simulink model "KeylessEntryArchitecture"  (R2024a)
settings: Solver=VariableStepAuto  StartTime=0.0  StopTime=10.0  RelTol=1e-3
settings Model: DataDictionary=Interfaces.sldd  Creator=The MathWorks, Inc.  LastModifiedBy=The MathWorks, Inc.
settings SolverCC: AlgebraicLoopSolver=TrustRegion
settings DebuggingCC: UnconnectedInputMsg=warning  UnconnectedOutputMsg=warning  UnconnectedLineMsg=warning  SymbolicDimsDataTypeCodeGenerationDiagnostic=none
settings ModelReferenceCC: EnableRefExpFcnMdlSchedulingChecks=on
settings RTWCC: GPUComputeCapability=3.5  DLArmComputeVersion=19.05

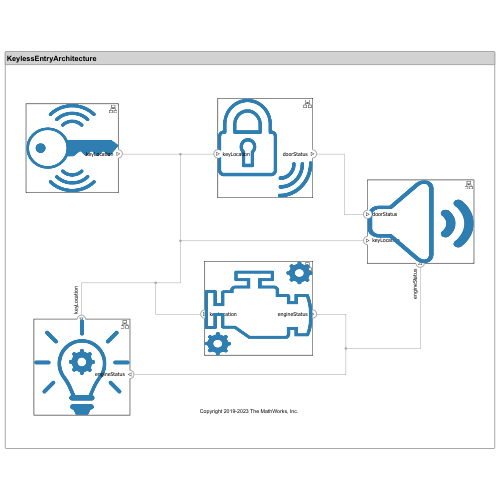
[thumbnail: Simulink's stored preview of the top-level diagram]
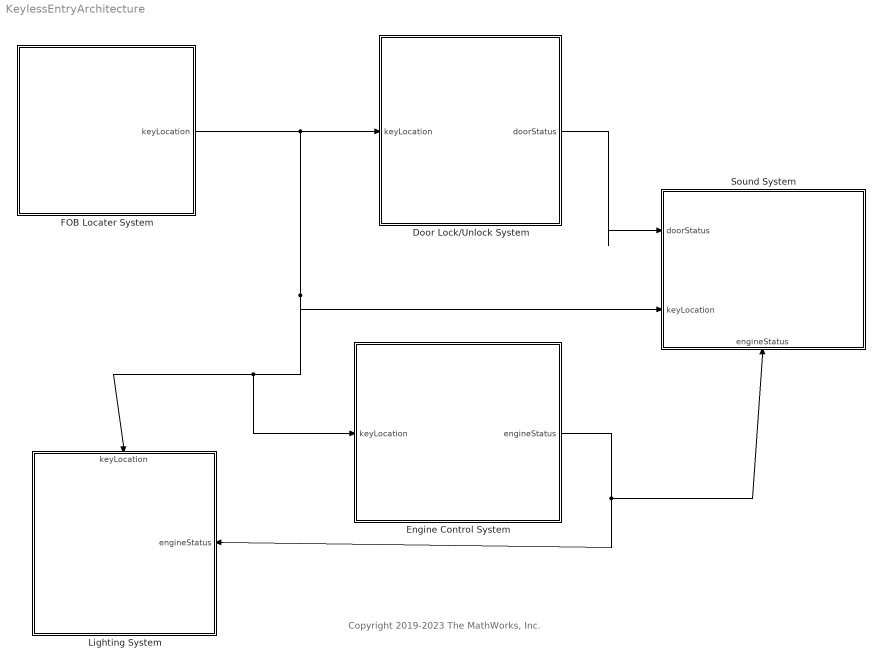
== system KeylessEntryArchitecture ==
  note: Copyright 2019-2023 The MathWorks, Inc.
  Door Lock/Unlock System : Subsystem
      settings: PortSchema="{\"entries\":[{\"content\":{\"headerSize\":26,\"margin\":15,\"minimumSpacing\":25,\"sides\":[{\"content\":{\"connectorIds\":[\"In1\"]},\"type\":\"ConnectorPlacement.EquallySpacedRectSide\",\"uuid\":\"159ee682-9fed-4fbb-9d94-5dba31d2910e\"},{\"content\":{\"connectorIds\":[\"Out1\"],\"side\":\"RIGHT\"},\"type\":\"ConnectorPlacement.EquallySpacedRectSide\",\"uuid\":\"29b28cc0-b170-4369-a93a-656923dab01a\"},{\"content\":{\"connectorIds\":[],\"side\":\"TOP\"},\"type\":\"ConnectorPlacement.EquallySpacedRectSide\",\"uuid\":\"ccfc0ebb-e385-4049-95f8-9f41f6dbc5fa\"}]},\"type\":\"ConnectorPlacement.EquallySpacedConnector\",\"uuid\":\"edbc9e1e-b6af-4ee7-9cbe-c6e12d5af40d\"}],\"packageUris\":[\"http://schema.mathworks.com/mf0/Connector/19700101\"],\"version\":\"1.0\"}"
      mask Display: image('door_lock_icon.png');
  Engine Control System : Subsystem
      settings: PortSchema="{\"entries\":[{\"content\":{\"headerSize\":26,\"margin\":15,\"minimumSpacing\":25,\"sides\":[{\"content\":{\"connectorIds\":[\"In1\"]},\"type\":\"ConnectorPlacement.EquallySpacedRectSide\",\"uuid\":\"159ee682-9fed-4fbb-9d94-5dba31d2910e\"},{\"content\":{\"connectorIds\":[\"Out1\"],\"side\":\"RIGHT\"},\"type\":\"ConnectorPlacement.EquallySpacedRectSide\",\"uuid\":\"29b28cc0-b170-4369-a93a-656923dab01a\"},{\"content\":{\"connectorIds\":[],\"side\":\"TOP\"},\"type\":\"ConnectorPlacement.EquallySpacedRectSide\",\"uuid\":\"ccfc0ebb-e385-4049-95f8-9f41f6dbc5fa\"}]},\"type\":\"ConnectorPlacement.EquallySpacedConnector\",\"uuid\":\"edbc9e1e-b6af-4ee7-9cbe-c6e12d5af40d\"}],\"packageUris\":[\"http://schema.mathworks.com/mf0/Connector/19700101\"],\"version\":\"1.0\"}"
      mask Display: image('engine_control_icon.png');
  FOB Locater System : Subsystem
      settings: PortSchema="{\"entries\":[{\"content\":{\"headerSize\":26,\"margin\":15,\"minimumSpacing\":25,\"sides\":[{\"content\":{\"connectorIds\":[]},\"type\":\"ConnectorPlacement.EquallySpacedRectSide\",\"uuid\":\"159ee682-9fed-4fbb-9d94-5dba31d2910e\"},{\"content\":{\"connectorIds\":[\"Out1\"],\"side\":\"RIGHT\"},\"type\":\"ConnectorPlacement.EquallySpacedRectSide\",\"uuid\":\"29b28cc0-b170-4369-a93a-656923dab01a\"},{\"content\":{\"connectorIds\":[],\"side\":\"TOP\"},\"type\":\"ConnectorPlacement.EquallySpacedRectSide\",\"uuid\":\"ccfc0ebb-e385-4049-95f8-9f41f6dbc5fa\"}]},\"type\":\"ConnectorPlacement.EquallySpacedConnector\",\"uuid\":\"edbc9e1e-b6af-4ee7-9cbe-c6e12d5af40d\"}],\"packageUris\":[\"http://schema.mathworks.com/mf0/Connector/19700101\"],\"version\":\"1.0\"}"
      mask Display: image('fob_locator_icon.png');
  Lighting System : Subsystem
      settings: PortSchema="{\"entries\":[{\"content\":{\"headerSize\":26,\"margin\":15,\"minimumSpacing\":25,\"sides\":[{\"content\":{\"connectorIds\":[]},\"type\":\"ConnectorPlacement.EquallySpacedRectSide\",\"uuid\":\"159ee682-9fed-4fbb-9d94-5dba31d2910e\"},{\"content\":{\"connectorIds\":[\"In2\"],\"side\":\"RIGHT\"},\"type\":\"ConnectorPlacement.EquallySpacedRectSide\",\"uuid\":\"29b28cc0-b170-4369-a93a-656923dab01a\"},{\"content\":{\"connectorIds\":[\"In1\"],\"side\":\"TOP\"},\"type\":\"ConnectorPlacement.EquallySpacedRectSide\",\"uuid\":\"ccfc0ebb-e385-4049-95f8-9f41f6dbc5fa\"}]},\"type\":\"ConnectorPlacement.EquallySpacedConnector\",\"uuid\":\"edbc9e1e-b6af-4ee7-9cbe-c6e12d5af40d\"}],\"packageUris\":[\"http://schema.mathworks.com/mf0/Connector/19700101\"],\"version\":\"1.0\"}"
      mask Display: image('lighting_system_icon.png');
  Sound System : Subsystem
      settings: PortSchema="{\"entries\":[{\"content\":{\"headerSize\":26,\"margin\":15,\"minimumSpacing\":25,\"sides\":[{\"content\":{\"connectorIds\":[\"In3\",\"In2\"]},\"type\":\"ConnectorPlacement.EquallySpacedRectSide\",\"uuid\":\"159ee682-9fed-4fbb-9d94-5dba31d2910e\"},{\"content\":{\"connectorIds\":[],\"side\":\"RIGHT\"},\"type\":\"ConnectorPlacement.EquallySpacedRectSide\",\"uuid\":\"29b28cc0-b170-4369-a93a-656923dab01a\"},{\"content\":{\"connectorIds\":[],\"side\":\"TOP\"},\"type\":\"ConnectorPlacement.EquallySpacedRectSide\",\"uuid\":\"ccfc0ebb-e385-4049-95f8-9f41f6dbc5fa\"},{\"content\":{\"connectorIds\":[\"In1\"],\"side\":\"BOTTOM\"},\"type\":\"ConnectorPlacement.EquallySpacedRectSide\",\"uuid\":\"874e8f25-aa17-4249-8800-ee0df902b395\"}]},\"type\":\"ConnectorPlacement.EquallySpacedConnector\",\"uuid\":\"edbc9e1e-b6af-4ee7-9cbe-c6e12d5af40d\"}],\"packageUris\":[\"http://schema.mathworks.com/mf0/Connector/19700101\"],\"version\":\"1.0\"}"
      mask Display: image('sound_system_icon.png');
  wires:
  FOB Locater System/1(keyLocation) -> Door Lock/Unlock System/1(keyLocation), Lighting System/1(keyLocation), Engine Control System/1(keyLocation), Sound System/2(keyLocation)
  Door Lock/Unlock System/1(doorStatus) -> Sound System/3(doorStatus)
  Engine Control System/1(engineStatus) -> Lighting System/2(engineStatus), Sound System/1(engineStatus)

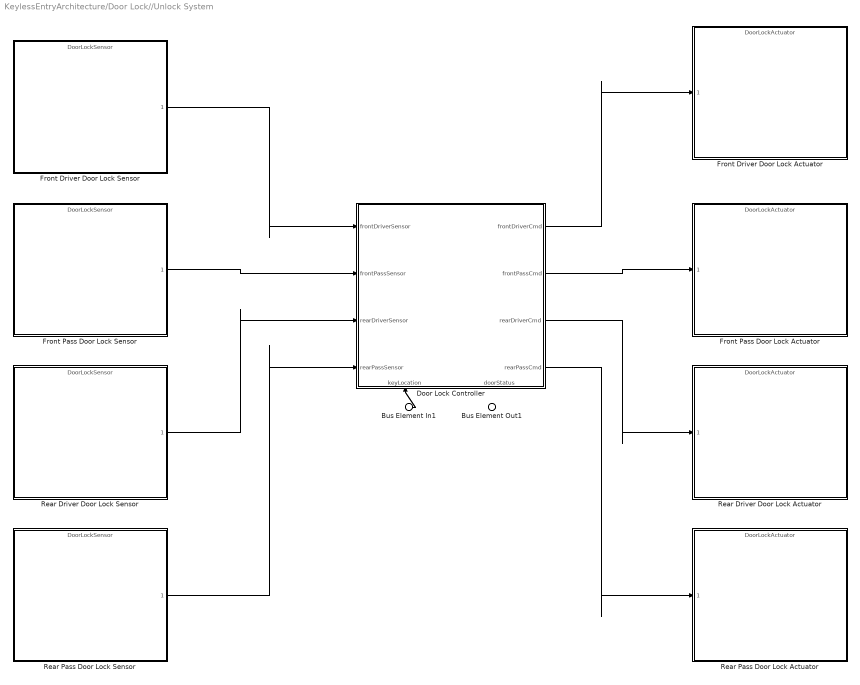
== system KeylessEntryArchitecture/Door Lock//Unlock System ==
  Bus Element In1 : Inport  PortName=keyLocation
  Door Lock Controller : Subsystem
      settings: PortSchema="{\"entries\":[{\"content\":{\"headerSize\":26,\"margin\":15,\"minimumSpacing\":25,\"sides\":[{\"content\":{\"connectorIds\":[\"In2\",\"In3\",\"In4\",\"In5\"]},\"type\":\"ConnectorPlacement.EquallySpacedRectSide\",\"uuid\":\"a0f82e88-5275-4bb9-87fe-a49bf19782cf\"},{\"content\":{\"connectorIds\":[\"Out1\",\"Out3\",\"Out4\",\"Out5\"],\"side\":\"RIGHT\"},\"type\":\"ConnectorPlacement.EquallySpacedRectSide\",\"uuid\":\"4b3945c4-3891-41a7-b741-bb467a4ccb5a\"},{\"content\":{\"connectorIds\":[],\"side\":\"TOP\"},\"type\":\"ConnectorPlacement.EquallySpacedRectSide\",\"uuid\":\"042b1b4e-e1cf-4b0e-a9d9-106bb99a7cf5\"},{\"content\":{\"connectorIds\":[\"In1\",\"Out2\"],\"side\":\"BOTTOM\"},\"type\":\"ConnectorPlacement.EquallySpacedRectSide\",\"uuid\":\"6aa53690-4f36-48a3-9490-70419d307c63\"}]},\"type\":\"ConnectorPlacement.EquallySpacedConnector\",\"uuid\":\"79d888da-39cf-4e1d-aa7b-1e8818e96d62\"}],\"packageUris\":[\"http://schema.mathworks.com/mf0/Connector/19700101\"],\"version\":\"1.0\"}"
  Front Driver Door Lock Actuator : ModelReference  ModelNameDialog=DoorLockActuator  SimulationMode=Normal  ModelReferenceVersion=8.5
      settings: PortSchema="{\"entries\":[{\"content\":{\"headerSize\":38,\"margin\":15,\"minimumSpacing\":25,\"sides\":[{\"content\":{\"connectorIds\":[\"In1\"]},\"type\":\"ConnectorPlacement.EquallySpacedRectSide\",\"uuid\":\"a0f82e88-5275-4bb9-87fe-a49bf19782cf\"},{\"content\":{\"connectorIds\":[],\"side\":\"RIGHT\"},\"type\":\"ConnectorPlacement.EquallySpacedRectSide\",\"uuid\":\"4b3945c4-3891-41a7-b741-bb467a4ccb5a\"},{\"content\":{\"connectorIds\":[],\"side\":\"TOP\"},\"type\":\"ConnectorPlacement.EquallySpacedRectSide\",\"uuid\":\"042b1b4e-e1cf-4b0e-a9d9-106bb99a7cf5\"}]},\"type\":\"ConnectorPlacement.EquallySpacedConnector\",\"uuid\":\"79d888da-39cf-4e1d-aa7b-1e8818e96d62\"}],\"packageUris\":[\"http://schema.mathworks.com/mf0/Connector/19700101\"],\"version\":\"1.0\"}"
  Front Driver Door Lock Sensor : ModelReference  ModelNameDialog=DoorLockSensor  SimulationMode=Normal  ModelReferenceVersion=8.5
      settings: PortSchema="{\"entries\":[{\"content\":{\"headerSize\":38,\"margin\":15,\"minimumSpacing\":25,\"sides\":[{\"content\":{\"connectorIds\":[]},\"type\":\"ConnectorPlacement.EquallySpacedRectSide\",\"uuid\":\"a0f82e88-5275-4bb9-87fe-a49bf19782cf\"},{\"content\":{\"connectorIds\":[\"Out1\"],\"side\":\"RIGHT\"},\"type\":\"ConnectorPlacement.EquallySpacedRectSide\",\"uuid\":\"4b3945c4-3891-41a7-b741-bb467a4ccb5a\"},{\"content\":{\"connectorIds\":[],\"side\":\"TOP\"},\"type\":\"ConnectorPlacement.EquallySpacedRectSide\",\"uuid\":\"042b1b4e-e1cf-4b0e-a9d9-106bb99a7cf5\"}]},\"type\":\"ConnectorPlacement.EquallySpacedConnector\",\"uuid\":\"79d888da-39cf-4e1d-aa7b-1e8818e96d62\"}],\"packageUris\":[\"http://schema.mathworks.com/mf0/Connector/19700101\"],\"version\":\"1.0\"}"
  Front Pass Door Lock Actuator : ModelReference  ModelNameDialog=DoorLockActuator  SimulationMode=Normal  ModelReferenceVersion=8.5
      settings: PortSchema="{\"entries\":[{\"content\":{\"headerSize\":38,\"margin\":15,\"minimumSpacing\":25,\"sides\":[{\"content\":{\"connectorIds\":[\"In1\"]},\"type\":\"ConnectorPlacement.EquallySpacedRectSide\",\"uuid\":\"a0f82e88-5275-4bb9-87fe-a49bf19782cf\"},{\"content\":{\"connectorIds\":[],\"side\":\"RIGHT\"},\"type\":\"ConnectorPlacement.EquallySpacedRectSide\",\"uuid\":\"4b3945c4-3891-41a7-b741-bb467a4ccb5a\"},{\"content\":{\"connectorIds\":[],\"side\":\"TOP\"},\"type\":\"ConnectorPlacement.EquallySpacedRectSide\",\"uuid\":\"042b1b4e-e1cf-4b0e-a9d9-106bb99a7cf5\"}]},\"type\":\"ConnectorPlacement.EquallySpacedConnector\",\"uuid\":\"79d888da-39cf-4e1d-aa7b-1e8818e96d62\"}],\"packageUris\":[\"http://schema.mathworks.com/mf0/Connector/19700101\"],\"version\":\"1.0\"}"
  Front Pass Door Lock Sensor : ModelReference  ModelNameDialog=DoorLockSensor  SimulationMode=Normal  ModelReferenceVersion=8.5
      settings: PortSchema="{\"entries\":[{\"content\":{\"headerSize\":38,\"margin\":15,\"minimumSpacing\":25,\"sides\":[{\"content\":{\"connectorIds\":[]},\"type\":\"ConnectorPlacement.EquallySpacedRectSide\",\"uuid\":\"a0f82e88-5275-4bb9-87fe-a49bf19782cf\"},{\"content\":{\"connectorIds\":[\"Out1\"],\"side\":\"RIGHT\"},\"type\":\"ConnectorPlacement.EquallySpacedRectSide\",\"uuid\":\"4b3945c4-3891-41a7-b741-bb467a4ccb5a\"},{\"content\":{\"connectorIds\":[],\"side\":\"TOP\"},\"type\":\"ConnectorPlacement.EquallySpacedRectSide\",\"uuid\":\"042b1b4e-e1cf-4b0e-a9d9-106bb99a7cf5\"}]},\"type\":\"ConnectorPlacement.EquallySpacedConnector\",\"uuid\":\"79d888da-39cf-4e1d-aa7b-1e8818e96d62\"}],\"packageUris\":[\"http://schema.mathworks.com/mf0/Connector/19700101\"],\"version\":\"1.0\"}"
  Rear Driver Door Lock Actuator : ModelReference  ModelNameDialog=DoorLockActuator  SimulationMode=Normal  ModelReferenceVersion=8.5
      settings: PortSchema="{\"entries\":[{\"content\":{\"headerSize\":38,\"margin\":15,\"minimumSpacing\":25,\"sides\":[{\"content\":{\"connectorIds\":[\"In1\"]},\"type\":\"ConnectorPlacement.EquallySpacedRectSide\",\"uuid\":\"a0f82e88-5275-4bb9-87fe-a49bf19782cf\"},{\"content\":{\"connectorIds\":[],\"side\":\"RIGHT\"},\"type\":\"ConnectorPlacement.EquallySpacedRectSide\",\"uuid\":\"4b3945c4-3891-41a7-b741-bb467a4ccb5a\"},{\"content\":{\"connectorIds\":[],\"side\":\"TOP\"},\"type\":\"ConnectorPlacement.EquallySpacedRectSide\",\"uuid\":\"042b1b4e-e1cf-4b0e-a9d9-106bb99a7cf5\"}]},\"type\":\"ConnectorPlacement.EquallySpacedConnector\",\"uuid\":\"79d888da-39cf-4e1d-aa7b-1e8818e96d62\"}],\"packageUris\":[\"http://schema.mathworks.com/mf0/Connector/19700101\"],\"version\":\"1.0\"}"
  Rear Driver Door Lock Sensor : ModelReference  ModelNameDialog=DoorLockSensor  SimulationMode=Normal  ModelReferenceVersion=8.5
      settings: PortSchema="{\"entries\":[{\"content\":{\"headerSize\":38,\"margin\":15,\"minimumSpacing\":25,\"sides\":[{\"content\":{\"connectorIds\":[]},\"type\":\"ConnectorPlacement.EquallySpacedRectSide\",\"uuid\":\"a0f82e88-5275-4bb9-87fe-a49bf19782cf\"},{\"content\":{\"connectorIds\":[\"Out1\"],\"side\":\"RIGHT\"},\"type\":\"ConnectorPlacement.EquallySpacedRectSide\",\"uuid\":\"4b3945c4-3891-41a7-b741-bb467a4ccb5a\"},{\"content\":{\"connectorIds\":[],\"side\":\"TOP\"},\"type\":\"ConnectorPlacement.EquallySpacedRectSide\",\"uuid\":\"042b1b4e-e1cf-4b0e-a9d9-106bb99a7cf5\"}]},\"type\":\"ConnectorPlacement.EquallySpacedConnector\",\"uuid\":\"79d888da-39cf-4e1d-aa7b-1e8818e96d62\"}],\"packageUris\":[\"http://schema.mathworks.com/mf0/Connector/19700101\"],\"version\":\"1.0\"}"
  Rear Pass Door Lock Actuator : ModelReference  ModelNameDialog=DoorLockActuator  SimulationMode=Normal  ModelReferenceVersion=8.5
      settings: PortSchema="{\"entries\":[{\"content\":{\"headerSize\":38,\"margin\":15,\"minimumSpacing\":25,\"sides\":[{\"content\":{\"connectorIds\":[\"In1\"]},\"type\":\"ConnectorPlacement.EquallySpacedRectSide\",\"uuid\":\"a0f82e88-5275-4bb9-87fe-a49bf19782cf\"},{\"content\":{\"connectorIds\":[],\"side\":\"RIGHT\"},\"type\":\"ConnectorPlacement.EquallySpacedRectSide\",\"uuid\":\"4b3945c4-3891-41a7-b741-bb467a4ccb5a\"},{\"content\":{\"connectorIds\":[],\"side\":\"TOP\"},\"type\":\"ConnectorPlacement.EquallySpacedRectSide\",\"uuid\":\"042b1b4e-e1cf-4b0e-a9d9-106bb99a7cf5\"}]},\"type\":\"ConnectorPlacement.EquallySpacedConnector\",\"uuid\":\"79d888da-39cf-4e1d-aa7b-1e8818e96d62\"}],\"packageUris\":[\"http://schema.mathworks.com/mf0/Connector/19700101\"],\"version\":\"1.0\"}"
  Rear Pass Door Lock Sensor : ModelReference  ModelNameDialog=DoorLockSensor  SimulationMode=Normal  ModelReferenceVersion=8.5
      settings: PortSchema="{\"entries\":[{\"content\":{\"headerSize\":38,\"margin\":15,\"minimumSpacing\":25,\"sides\":[{\"content\":{\"connectorIds\":[]},\"type\":\"ConnectorPlacement.EquallySpacedRectSide\",\"uuid\":\"a0f82e88-5275-4bb9-87fe-a49bf19782cf\"},{\"content\":{\"connectorIds\":[\"Out1\"],\"side\":\"RIGHT\"},\"type\":\"ConnectorPlacement.EquallySpacedRectSide\",\"uuid\":\"4b3945c4-3891-41a7-b741-bb467a4ccb5a\"},{\"content\":{\"connectorIds\":[],\"side\":\"TOP\"},\"type\":\"ConnectorPlacement.EquallySpacedRectSide\",\"uuid\":\"042b1b4e-e1cf-4b0e-a9d9-106bb99a7cf5\"}]},\"type\":\"ConnectorPlacement.EquallySpacedConnector\",\"uuid\":\"79d888da-39cf-4e1d-aa7b-1e8818e96d62\"}],\"packageUris\":[\"http://schema.mathworks.com/mf0/Connector/19700101\"],\"version\":\"1.0\"}"
  Bus Element Out1 : Outport  PortName=doorStatus
  wires:
  Front Driver Door Lock Sensor/1 -> Door Lock Controller/2(frontDriverSensor)
  Front Pass Door Lock Sensor/1 -> Door Lock Controller/3(frontPassSensor)
  Rear Driver Door Lock Sensor/1 -> Door Lock Controller/4(rearDriverSensor)
  Rear Pass Door Lock Sensor/1 -> Door Lock Controller/5(rearPassSensor)
  Door Lock Controller/1(frontDriverCmd) -> Front Driver Door Lock Actuator/1
  Door Lock Controller/3(frontPassCmd) -> Front Pass Door Lock Actuator/1
  Door Lock Controller/4(rearDriverCmd) -> Rear Driver Door Lock Actuator/1
  Door Lock Controller/5(rearPassCmd) -> Rear Pass Door Lock Actuator/1
  Bus Element In1/1 -> Door Lock Controller/1(keyLocation)

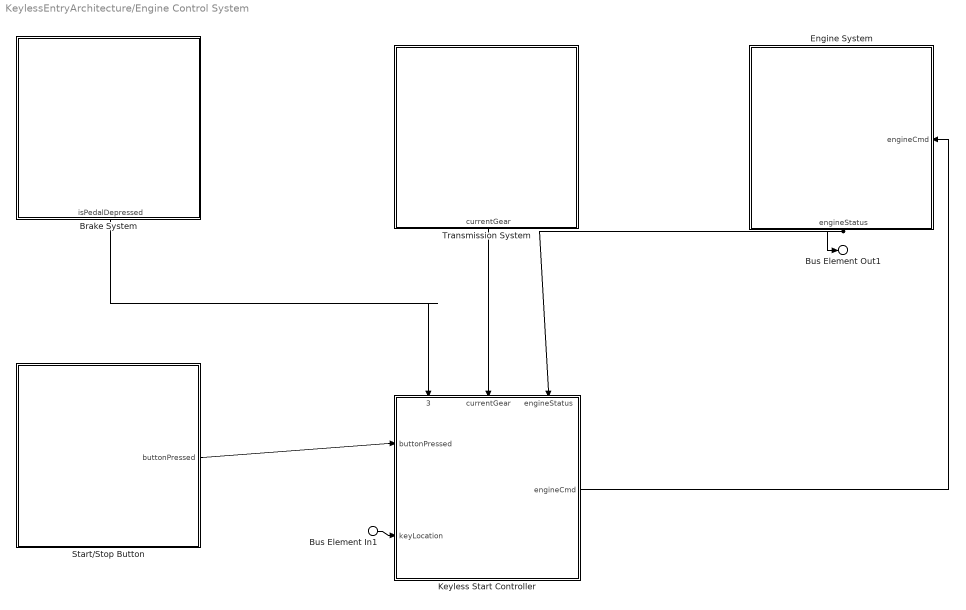
== system KeylessEntryArchitecture/Engine Control System ==
  Bus Element In1 : Inport  PortName=keyLocation
  Brake System : Subsystem
      settings: PortSchema="{\"entries\":[{\"content\":{\"headerSize\":26,\"margin\":15,\"minimumSpacing\":25,\"sides\":[{\"content\":{\"connectorIds\":[]},\"type\":\"ConnectorPlacement.EquallySpacedRectSide\",\"uuid\":\"a0f82e88-5275-4bb9-87fe-a49bf19782cf\"},{\"content\":{\"connectorIds\":[],\"side\":\"RIGHT\"},\"type\":\"ConnectorPlacement.EquallySpacedRectSide\",\"uuid\":\"4b3945c4-3891-41a7-b741-bb467a4ccb5a\"},{\"content\":{\"connectorIds\":[],\"side\":\"TOP\"},\"type\":\"ConnectorPlacement.EquallySpacedRectSide\",\"uuid\":\"042b1b4e-e1cf-4b0e-a9d9-106bb99a7cf5\"},{\"content\":{\"connectorIds\":[\"Out1\"],\"side\":\"BOTTOM\"},\"type\":\"ConnectorPlacement.EquallySpacedRectSide\",\"uuid\":\"2c1eff0a-c33a-441c-bf29-8810011e62b1\"}]},\"type\":\"ConnectorPlacement.EquallySpacedConnector\",\"uuid\":\"79d888da-39cf-4e1d-aa7b-1e8818e96d62\"}],\"packageUris\":[\"http://schema.mathworks.com/mf0/Connector/19700101\"],\"version\":\"1.0\"}"
  Engine System : Subsystem
      settings: PortSchema="{\"entries\":[{\"content\":{\"headerSize\":26,\"margin\":15,\"minimumSpacing\":25,\"sides\":[{\"content\":{\"connectorIds\":[]},\"type\":\"ConnectorPlacement.EquallySpacedRectSide\",\"uuid\":\"a0f82e88-5275-4bb9-87fe-a49bf19782cf\"},{\"content\":{\"connectorIds\":[\"In1\"],\"side\":\"RIGHT\"},\"type\":\"ConnectorPlacement.EquallySpacedRectSide\",\"uuid\":\"4b3945c4-3891-41a7-b741-bb467a4ccb5a\"},{\"content\":{\"connectorIds\":[],\"side\":\"TOP\"},\"type\":\"ConnectorPlacement.EquallySpacedRectSide\",\"uuid\":\"042b1b4e-e1cf-4b0e-a9d9-106bb99a7cf5\"},{\"content\":{\"connectorIds\":[\"Out1\"],\"side\":\"BOTTOM\"},\"type\":\"ConnectorPlacement.EquallySpacedRectSide\",\"uuid\":\"0362089f-4f80-4409-9348-df11b302b3ca\"}]},\"type\":\"ConnectorPlacement.EquallySpacedConnector\",\"uuid\":\"79d888da-39cf-4e1d-aa7b-1e8818e96d62\"}],\"packageUris\":[\"http://schema.mathworks.com/mf0/Connector/19700101\"],\"version\":\"1.0\"}"
  Keyless Start Controller : Subsystem
      settings: PortSchema="{\"entries\":[{\"content\":{\"headerSize\":26,\"margin\":15,\"minimumSpacing\":25,\"sides\":[{\"content\":{\"connectorIds\":[\"In1\",\"In2\"]},\"type\":\"ConnectorPlacement.EquallySpacedRectSide\",\"uuid\":\"a0f82e88-5275-4bb9-87fe-a49bf19782cf\"},{\"content\":{\"connectorIds\":[\"Out1\"],\"side\":\"RIGHT\"},\"type\":\"ConnectorPlacement.EquallySpacedRectSide\",\"uuid\":\"4b3945c4-3891-41a7-b741-bb467a4ccb5a\"},{\"content\":{\"connectorIds\":[\"In3\",\"In4\",\"In5\"],\"side\":\"TOP\"},\"type\":\"ConnectorPlacement.EquallySpacedRectSide\",\"uuid\":\"042b1b4e-e1cf-4b0e-a9d9-106bb99a7cf5\"}]},\"type\":\"ConnectorPlacement.EquallySpacedConnector\",\"uuid\":\"79d888da-39cf-4e1d-aa7b-1e8818e96d62\"}],\"packageUris\":[\"http://schema.mathworks.com/mf0/Connector/19700101\"],\"version\":\"1.0\"}"
  Start/Stop Button : Subsystem
      settings: PortSchema="{\"entries\":[{\"content\":{\"headerSize\":26,\"margin\":15,\"minimumSpacing\":25,\"sides\":[{\"content\":{\"connectorIds\":[]},\"type\":\"ConnectorPlacement.EquallySpacedRectSide\",\"uuid\":\"a0f82e88-5275-4bb9-87fe-a49bf19782cf\"},{\"content\":{\"connectorIds\":[\"Out1\"],\"side\":\"RIGHT\"},\"type\":\"ConnectorPlacement.EquallySpacedRectSide\",\"uuid\":\"4b3945c4-3891-41a7-b741-bb467a4ccb5a\"},{\"content\":{\"connectorIds\":[],\"side\":\"TOP\"},\"type\":\"ConnectorPlacement.EquallySpacedRectSide\",\"uuid\":\"042b1b4e-e1cf-4b0e-a9d9-106bb99a7cf5\"}]},\"type\":\"ConnectorPlacement.EquallySpacedConnector\",\"uuid\":\"79d888da-39cf-4e1d-aa7b-1e8818e96d62\"}],\"packageUris\":[\"http://schema.mathworks.com/mf0/Connector/19700101\"],\"version\":\"1.0\"}"
  Transmission System : Subsystem
      settings: PortSchema="{\"entries\":[{\"content\":{\"headerSize\":26,\"margin\":15,\"minimumSpacing\":25,\"sides\":[{\"content\":{\"connectorIds\":[]},\"type\":\"ConnectorPlacement.EquallySpacedRectSide\",\"uuid\":\"a0f82e88-5275-4bb9-87fe-a49bf19782cf\"},{\"content\":{\"connectorIds\":[],\"side\":\"RIGHT\"},\"type\":\"ConnectorPlacement.EquallySpacedRectSide\",\"uuid\":\"4b3945c4-3891-41a7-b741-bb467a4ccb5a\"},{\"content\":{\"connectorIds\":[],\"side\":\"TOP\"},\"type\":\"ConnectorPlacement.EquallySpacedRectSide\",\"uuid\":\"042b1b4e-e1cf-4b0e-a9d9-106bb99a7cf5\"},{\"content\":{\"connectorIds\":[\"Out1\"],\"side\":\"BOTTOM\"},\"type\":\"ConnectorPlacement.EquallySpacedRectSide\",\"uuid\":\"217a1e67-16b0-4a07-be4d-bf369191c717\"}]},\"type\":\"ConnectorPlacement.EquallySpacedConnector\",\"uuid\":\"79d888da-39cf-4e1d-aa7b-1e8818e96d62\"}],\"packageUris\":[\"http://schema.mathworks.com/mf0/Connector/19700101\"],\"version\":\"1.0\"}"
  Bus Element Out1 : Outport  PortName=engineStatus
  wires:
  Brake System/1(isPedalDepressed) -> Keyless Start Controller/3(isPedalDepressed)
  Transmission System/1(currentGear) -> Keyless Start Controller/4(currentGear)
  Engine System/1(engineStatus) -> Keyless Start Controller/5(engineStatus), Bus Element Out1/1
  Start/Stop Button/1(buttonPressed) -> Keyless Start Controller/1(buttonPressed)
  Keyless Start Controller/1(engineCmd) -> Engine System/1(engineCmd)
  Bus Element In1/1 -> Keyless Start Controller/2(keyLocation)

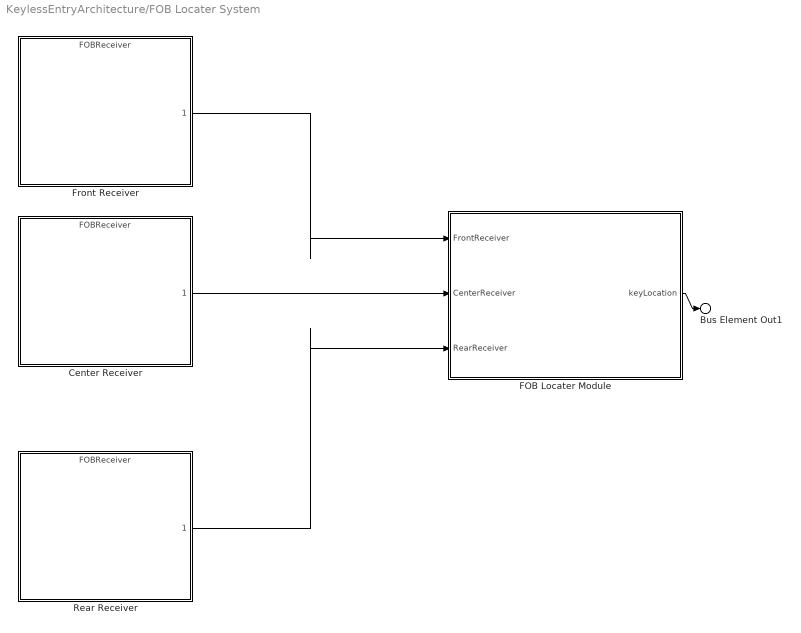
== system KeylessEntryArchitecture/FOB Locater System ==
  Center Receiver : ModelReference  ModelNameDialog=FOBReceiver  SimulationMode=Normal  ModelReferenceVersion=8.6
      settings: PortSchema="{\"entries\":[{\"content\":{\"headerSize\":38,\"margin\":15,\"minimumSpacing\":25,\"sides\":[{\"content\":{\"connectorIds\":[]},\"type\":\"ConnectorPlacement.EquallySpacedRectSide\",\"uuid\":\"a0f82e88-5275-4bb9-87fe-a49bf19782cf\"},{\"content\":{\"connectorIds\":[\"Out1\"],\"side\":\"RIGHT\"},\"type\":\"ConnectorPlacement.EquallySpacedRectSide\",\"uuid\":\"4b3945c4-3891-41a7-b741-bb467a4ccb5a\"},{\"content\":{\"connectorIds\":[],\"side\":\"TOP\"},\"type\":\"ConnectorPlacement.EquallySpacedRectSide\",\"uuid\":\"042b1b4e-e1cf-4b0e-a9d9-106bb99a7cf5\"}]},\"type\":\"ConnectorPlacement.EquallySpacedConnector\",\"uuid\":\"79d888da-39cf-4e1d-aa7b-1e8818e96d62\"}],\"packageUris\":[\"http://schema.mathworks.com/mf0/Connector/19700101\"],\"version\":\"1.0\"}"
  FOB Locater Module : Subsystem
      settings: PortSchema="{\"entries\":[{\"content\":{\"headerSize\":26,\"margin\":15,\"minimumSpacing\":25,\"sides\":[{\"content\":{\"connectorIds\":[\"In1\",\"In2\",\"In3\"]},\"type\":\"ConnectorPlacement.EquallySpacedRectSide\",\"uuid\":\"a0f82e88-5275-4bb9-87fe-a49bf19782cf\"},{\"content\":{\"connectorIds\":[\"Out1\"],\"side\":\"RIGHT\"},\"type\":\"ConnectorPlacement.EquallySpacedRectSide\",\"uuid\":\"4b3945c4-3891-41a7-b741-bb467a4ccb5a\"},{\"content\":{\"connectorIds\":[],\"side\":\"TOP\"},\"type\":\"ConnectorPlacement.EquallySpacedRectSide\",\"uuid\":\"042b1b4e-e1cf-4b0e-a9d9-106bb99a7cf5\"}]},\"type\":\"ConnectorPlacement.EquallySpacedConnector\",\"uuid\":\"79d888da-39cf-4e1d-aa7b-1e8818e96d62\"}],\"packageUris\":[\"http://schema.mathworks.com/mf0/Connector/19700101\"],\"version\":\"1.0\"}"
  Front Receiver : ModelReference  ModelNameDialog=FOBReceiver  SimulationMode=Normal  ModelReferenceVersion=8.6
      settings: PortSchema="{\"entries\":[{\"content\":{\"headerSize\":38,\"margin\":15,\"minimumSpacing\":25,\"sides\":[{\"content\":{\"connectorIds\":[]},\"type\":\"ConnectorPlacement.EquallySpacedRectSide\",\"uuid\":\"a0f82e88-5275-4bb9-87fe-a49bf19782cf\"},{\"content\":{\"connectorIds\":[\"Out1\"],\"side\":\"RIGHT\"},\"type\":\"ConnectorPlacement.EquallySpacedRectSide\",\"uuid\":\"4b3945c4-3891-41a7-b741-bb467a4ccb5a\"},{\"content\":{\"connectorIds\":[],\"side\":\"TOP\"},\"type\":\"ConnectorPlacement.EquallySpacedRectSide\",\"uuid\":\"042b1b4e-e1cf-4b0e-a9d9-106bb99a7cf5\"}]},\"type\":\"ConnectorPlacement.EquallySpacedConnector\",\"uuid\":\"79d888da-39cf-4e1d-aa7b-1e8818e96d62\"}],\"packageUris\":[\"http://schema.mathworks.com/mf0/Connector/19700101\"],\"version\":\"1.0\"}"
  Rear Receiver : ModelReference  ModelNameDialog=FOBReceiver  SimulationMode=Normal  ModelReferenceVersion=8.6
      settings: PortSchema="{\"entries\":[{\"content\":{\"headerSize\":38,\"margin\":15,\"minimumSpacing\":25,\"sides\":[{\"content\":{\"connectorIds\":[]},\"type\":\"ConnectorPlacement.EquallySpacedRectSide\",\"uuid\":\"a0f82e88-5275-4bb9-87fe-a49bf19782cf\"},{\"content\":{\"connectorIds\":[\"Out1\"],\"side\":\"RIGHT\"},\"type\":\"ConnectorPlacement.EquallySpacedRectSide\",\"uuid\":\"4b3945c4-3891-41a7-b741-bb467a4ccb5a\"},{\"content\":{\"connectorIds\":[],\"side\":\"TOP\"},\"type\":\"ConnectorPlacement.EquallySpacedRectSide\",\"uuid\":\"042b1b4e-e1cf-4b0e-a9d9-106bb99a7cf5\"}]},\"type\":\"ConnectorPlacement.EquallySpacedConnector\",\"uuid\":\"79d888da-39cf-4e1d-aa7b-1e8818e96d62\"}],\"packageUris\":[\"http://schema.mathworks.com/mf0/Connector/19700101\"],\"version\":\"1.0\"}"
  Bus Element Out1 : Outport  PortName=keyLocation
  wires:
  FOB Locater Module/1(keyLocation) -> Bus Element Out1/1
  Front Receiver/1 -> FOB Locater Module/1(FrontReceiver)
  Center Receiver/1 -> FOB Locater Module/2(CenterReceiver)
  Rear Receiver/1 -> FOB Locater Module/3(RearReceiver)

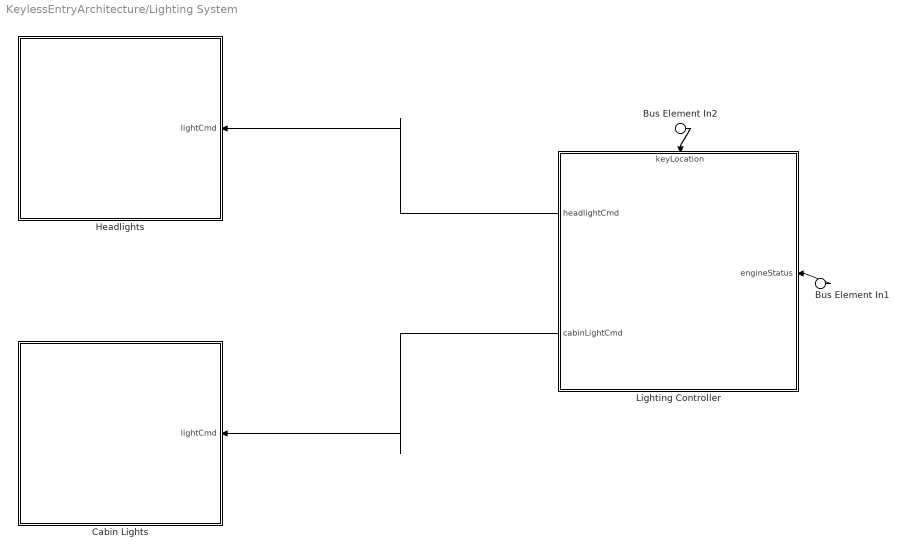
== system KeylessEntryArchitecture/Lighting System ==
  Bus Element In2 : Inport  PortName=keyLocation
  Bus Element In1 : Inport  Port=2  PortName=engineStatus
  Cabin Lights : Subsystem
      settings: PortSchema="{\"entries\":[{\"content\":{\"headerSize\":26,\"margin\":15,\"minimumSpacing\":25,\"sides\":[{\"content\":{\"connectorIds\":[]},\"type\":\"ConnectorPlacement.EquallySpacedRectSide\",\"uuid\":\"a0f82e88-5275-4bb9-87fe-a49bf19782cf\"},{\"content\":{\"connectorIds\":[\"In1\"],\"side\":\"RIGHT\"},\"type\":\"ConnectorPlacement.EquallySpacedRectSide\",\"uuid\":\"4b3945c4-3891-41a7-b741-bb467a4ccb5a\"},{\"content\":{\"connectorIds\":[],\"side\":\"TOP\"},\"type\":\"ConnectorPlacement.EquallySpacedRectSide\",\"uuid\":\"042b1b4e-e1cf-4b0e-a9d9-106bb99a7cf5\"}]},\"type\":\"ConnectorPlacement.EquallySpacedConnector\",\"uuid\":\"79d888da-39cf-4e1d-aa7b-1e8818e96d62\"}],\"packageUris\":[\"http://schema.mathworks.com/mf0/Connector/19700101\"],\"version\":\"1.0\"}"
  Headlights : Subsystem
      settings: PortSchema="{\"entries\":[{\"content\":{\"headerSize\":26,\"margin\":15,\"minimumSpacing\":25,\"sides\":[{\"content\":{\"connectorIds\":[]},\"type\":\"ConnectorPlacement.EquallySpacedRectSide\",\"uuid\":\"a0f82e88-5275-4bb9-87fe-a49bf19782cf\"},{\"content\":{\"connectorIds\":[\"In1\"],\"side\":\"RIGHT\"},\"type\":\"ConnectorPlacement.EquallySpacedRectSide\",\"uuid\":\"4b3945c4-3891-41a7-b741-bb467a4ccb5a\"},{\"content\":{\"connectorIds\":[],\"side\":\"TOP\"},\"type\":\"ConnectorPlacement.EquallySpacedRectSide\",\"uuid\":\"042b1b4e-e1cf-4b0e-a9d9-106bb99a7cf5\"}]},\"type\":\"ConnectorPlacement.EquallySpacedConnector\",\"uuid\":\"79d888da-39cf-4e1d-aa7b-1e8818e96d62\"}],\"packageUris\":[\"http://schema.mathworks.com/mf0/Connector/19700101\"],\"version\":\"1.0\"}"
  Lighting Controller : Subsystem
      settings: PortSchema="{\"entries\":[{\"content\":{\"headerSize\":26,\"margin\":15,\"minimumSpacing\":25,\"sides\":[{\"content\":{\"connectorIds\":[\"Out1\",\"Out2\"]},\"type\":\"ConnectorPlacement.EquallySpacedRectSide\",\"uuid\":\"a0f82e88-5275-4bb9-87fe-a49bf19782cf\"},{\"content\":{\"connectorIds\":[\"In1\"],\"side\":\"RIGHT\"},\"type\":\"ConnectorPlacement.EquallySpacedRectSide\",\"uuid\":\"4b3945c4-3891-41a7-b741-bb467a4ccb5a\"},{\"content\":{\"connectorIds\":[\"In2\"],\"side\":\"TOP\"},\"type\":\"ConnectorPlacement.EquallySpacedRectSide\",\"uuid\":\"042b1b4e-e1cf-4b0e-a9d9-106bb99a7cf5\"}]},\"type\":\"ConnectorPlacement.EquallySpacedConnector\",\"uuid\":\"79d888da-39cf-4e1d-aa7b-1e8818e96d62\"}],\"packageUris\":[\"http://schema.mathworks.com/mf0/Connector/19700101\"],\"version\":\"1.0\"}"
  wires:
  Bus Element In2/1 -> Lighting Controller/2(keyLocation)
  Bus Element In1/1 -> Lighting Controller/1(engineStatus)
  Lighting Controller/1(headlightCmd) -> Headlights/1(lightCmd)
  Lighting Controller/2(cabinLightCmd) -> Cabin Lights/1(lightCmd)

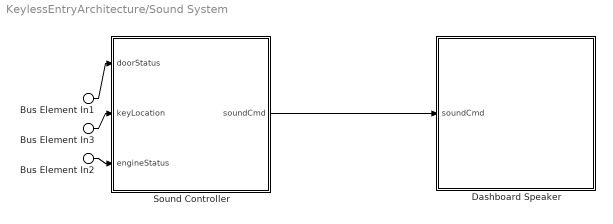
== system KeylessEntryArchitecture/Sound System ==
  Bus Element In2 : Inport  PortName=engineStatus
  Bus Element In3 : Inport  Port=2  PortName=keyLocation
  Bus Element In1 : Inport  Port=3  PortName=doorStatus
  Dashboard Speaker : Subsystem
      settings: PortSchema="{\"entries\":[{\"content\":{\"headerSize\":26,\"margin\":15,\"minimumSpacing\":25,\"sides\":[{\"content\":{\"connectorIds\":[\"In1\"]},\"type\":\"ConnectorPlacement.EquallySpacedRectSide\",\"uuid\":\"a0f82e88-5275-4bb9-87fe-a49bf19782cf\"},{\"content\":{\"connectorIds\":[],\"side\":\"RIGHT\"},\"type\":\"ConnectorPlacement.EquallySpacedRectSide\",\"uuid\":\"4b3945c4-3891-41a7-b741-bb467a4ccb5a\"},{\"content\":{\"connectorIds\":[],\"side\":\"TOP\"},\"type\":\"ConnectorPlacement.EquallySpacedRectSide\",\"uuid\":\"042b1b4e-e1cf-4b0e-a9d9-106bb99a7cf5\"}]},\"type\":\"ConnectorPlacement.EquallySpacedConnector\",\"uuid\":\"79d888da-39cf-4e1d-aa7b-1e8818e96d62\"}],\"packageUris\":[\"http://schema.mathworks.com/mf0/Connector/19700101\"],\"version\":\"1.0\"}"
  Sound Controller : Subsystem
      settings: PortSchema="{\"entries\":[{\"content\":{\"headerSize\":26,\"margin\":15,\"minimumSpacing\":25,\"sides\":[{\"content\":{\"connectorIds\":[\"In1\",\"In2\",\"In3\"]},\"type\":\"ConnectorPlacement.EquallySpacedRectSide\",\"uuid\":\"a0f82e88-5275-4bb9-87fe-a49bf19782cf\"},{\"content\":{\"connectorIds\":[\"Out1\"],\"side\":\"RIGHT\"},\"type\":\"ConnectorPlacement.EquallySpacedRectSide\",\"uuid\":\"4b3945c4-3891-41a7-b741-bb467a4ccb5a\"},{\"content\":{\"connectorIds\":[],\"side\":\"TOP\"},\"type\":\"ConnectorPlacement.EquallySpacedRectSide\",\"uuid\":\"042b1b4e-e1cf-4b0e-a9d9-106bb99a7cf5\"}]},\"type\":\"ConnectorPlacement.EquallySpacedConnector\",\"uuid\":\"79d888da-39cf-4e1d-aa7b-1e8818e96d62\"}],\"packageUris\":[\"http://schema.mathworks.com/mf0/Connector/19700101\"],\"version\":\"1.0\"}"
  wires:
  Sound Controller/1(soundCmd) -> Dashboard Speaker/1(soundCmd)
  Bus Element In1/1 -> Sound Controller/1(doorStatus)
  Bus Element In3/1 -> Sound Controller/2(keyLocation)
  Bus Element In2/1 -> Sound Controller/3(engineStatus)

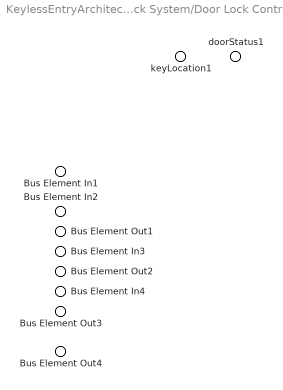
== system KeylessEntryArchitecture/Door Lock//Unlock System/Door Lock Controller ==
  keyLocation1 : Inport  PortName=keyLocation
  Bus Element In1 : Inport  Port=2  PortName=frontDriverSensor
  Bus Element In2 : Inport  Port=3  PortName=frontPassSensor
  Bus Element In3 : Inport  Port=4  PortName=rearDriverSensor
  Bus Element In4 : Inport  Port=5  PortName=rearPassSensor
  Bus Element Out1 : Outport  PortName=frontDriverCmd
  doorStatus1 : Outport  Port=2  PortName=doorStatus
  Bus Element Out2 : Outport  Port=3  PortName=frontPassCmd
  Bus Element Out3 : Outport  Port=4  PortName=rearDriverCmd
  Bus Element Out4 : Outport  Port=5  PortName=rearPassCmd

== system KeylessEntryArchitecture/Engine Control System/Brake System ==
  Bus Element Out1 : Outport  PortName=isPedalDepressed

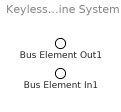
== system KeylessEntryArchitecture/Engine Control System/Engine System ==
  Bus Element In1 : Inport  PortName=engineCmd
  Bus Element Out1 : Outport  PortName=engineStatus

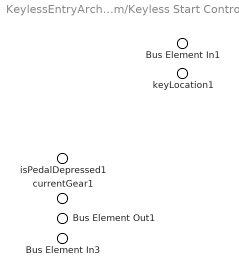
== system KeylessEntryArchitecture/Engine Control System/Keyless Start Controller ==
  Bus Element In1 : Inport  PortName=buttonPressed
  keyLocation1 : Inport  Port=2  PortName=keyLocation
  isPedalDepressed1 : Inport  Port=3  PortName=isPedalDepressed
  currentGear1 : Inport  Port=4  PortName=currentGear
  Bus Element In3 : Inport  Port=5  PortName=engineStatus
  Bus Element Out1 : Outport  PortName=engineCmd

== system KeylessEntryArchitecture/Engine Control System/Start//Stop Button ==
  Bus Element Out1 : Outport  PortName=buttonPressed

== system KeylessEntryArchitecture/Engine Control System/Transmission System ==
  Bus Element Out1 : Outport  PortName=currentGear

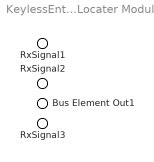
== system KeylessEntryArchitecture/FOB Locater System/FOB Locater Module ==
  RxSignal1 : Inport  PortName=FrontReceiver
  RxSignal2 : Inport  Port=2  PortName=CenterReceiver
  RxSignal3 : Inport  Port=3  PortName=RearReceiver
  Bus Element Out1 : Outport  PortName=keyLocation

== system KeylessEntryArchitecture/Lighting System/Cabin Lights ==
  lightCmd1 : Inport  PortName=lightCmd

== system KeylessEntryArchitecture/Lighting System/Headlights ==
  Bus Element In1 : Inport  PortName=lightCmd

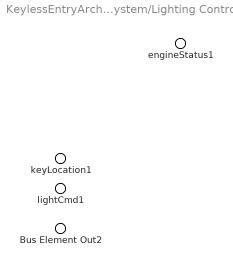
== system KeylessEntryArchitecture/Lighting System/Lighting Controller ==
  engineStatus1 : Inport  PortName=engineStatus
  keyLocation1 : Inport  Port=2  PortName=keyLocation
  lightCmd1 : Outport  PortName=headlightCmd
  Bus Element Out2 : Outport  Port=2  PortName=cabinLightCmd

== system KeylessEntryArchitecture/Sound System/Dashboard Speaker ==
  Bus Element In1 : Inport  PortName=soundCmd

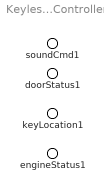
== system KeylessEntryArchitecture/Sound System/Sound Controller ==
  doorStatus1 : Inport  PortName=doorStatus
  keyLocation1 : Inport  Port=2  PortName=keyLocation
  engineStatus1 : Inport  Port=3  PortName=engineStatus
  soundCmd1 : Outport  PortName=soundCmd
